simulink model "KF_Model_Div_Fixed"  (R2024b)
settings: Solver=FixedStepAuto  StartTime=0.0  StopTime=0.0025  FixedStep=5e-6  RelTol=1e-3
libraries: dspsrcs4 x3
settings Model: Creator=bzwan  LastModifiedBy=bzwan
settings OptimizationCC: UseDivisionForNetSlopeComputation=on
settings DebuggingCC: SignalRangeChecking=warning
settings HardwareCC: ProdBitPerPointer=32  ProdBitPerSizeT=32  ProdBitPerPtrDiffT=32  ProdLargestAtomicFloat=None  ProdIntDivRoundTo=Undefined  ProdEndianess=Unspecified  ProdWordSize=32  ProdHWDeviceType=ASIC/FPGA->ASIC/FPGA  TargetBitPerPointer=64  TargetBitPerSizeT=64  TargetBitPerPtrDiffT=64  TargetLongLongMode=on  TargetIntDivRoundTo=Zero  TargetEndianess=LittleEndian  TargetWordSize=64  TargetHWDeviceType=Custom Processor->MATLAB Host Computer  ProdEqTarget=off

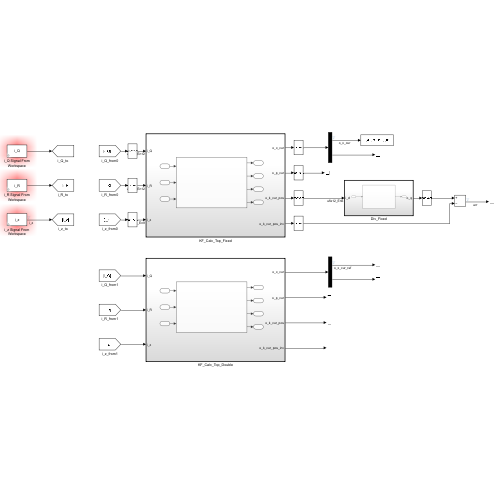
[thumbnail: Simulink's stored preview of the top-level diagram]
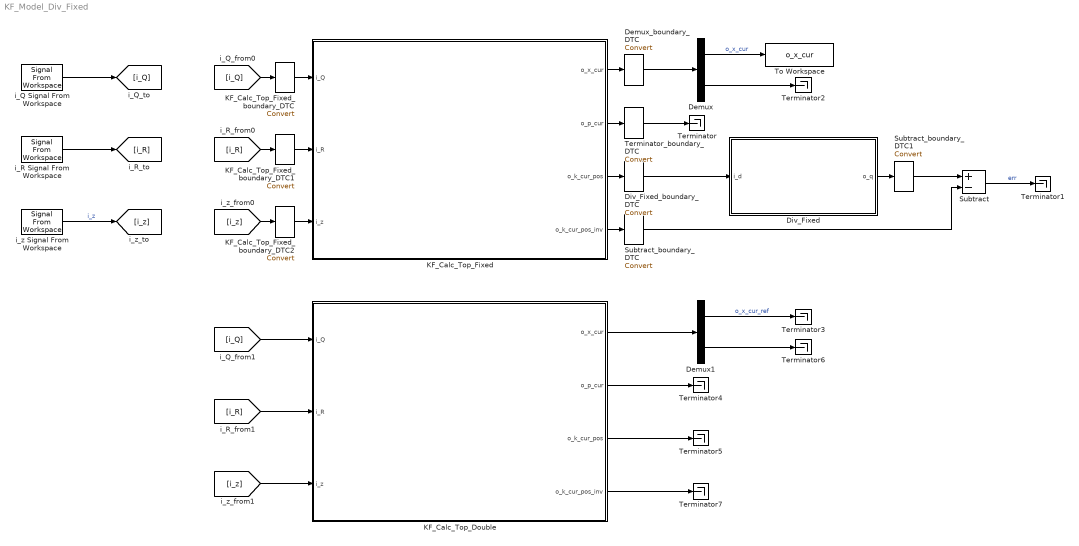
== system KF_Model_Div_Fixed ==
  Demux : Demux  Outputs=2
  Demux1 : Demux  Outputs=2
  Demux_boundary_DTC : DataTypeConversion
  Div_Fixed : Subsystem  TreatAsAtomicUnit=on  SystemSampleTime=1/10000
  Div_Fixed_boundary_DTC : DataTypeConversion
  KF_Calc_Top_Double : Subsystem  TreatAsAtomicUnit=on  SystemSampleTime=1/10000
  KF_Calc_Top_Fixed : Subsystem  TreatAsAtomicUnit=on  SystemSampleTime=1/10000
  KF_Calc_Top_Fixed_boundary_DTC : DataTypeConversion
  KF_Calc_Top_Fixed_boundary_DTC1 : DataTypeConversion
  KF_Calc_Top_Fixed_boundary_DTC2 : DataTypeConversion
  Subtract : Sum  Inputs=+-
  Subtract_boundary_DTC : DataTypeConversion
  Subtract_boundary_DTC1 : DataTypeConversion
  Terminator{,1..7} (8 alike) : Terminator
  Terminator_boundary_DTC : DataTypeConversion
  To Workspace : ToWorkspace  VariableName=o_x_cur  SaveFormat=Structure  SampleTime=-1
  i_Q Signal From Workspace : dspsrcs4/Signal From Workspace  X=i_Q  Ts=1/10000  nsamps=1  OutputAfterFinalValue=Cyclic repetition  ignoreOrWarnInputAndFrameLengths=off  OutputFrames=off
  i_R Signal From Workspace : dspsrcs4/Signal From Workspace  X=i_R  Ts=1/10000  nsamps=1  OutputAfterFinalValue=Cyclic repetition  ignoreOrWarnInputAndFrameLengths=off  OutputFrames=off
  i_z Signal From Workspace : dspsrcs4/Signal From Workspace  X=i_z  Ts=1/10000  nsamps=1  OutputAfterFinalValue=Cyclic repetition  ignoreOrWarnInputAndFrameLengths=off  OutputFrames=off
  wires:
  KF_Calc_Top_Double/1(o_x_cur) -> Demux1/1
  KF_Calc_Top_Double/2(o_p_cur) -> Terminator4/1
  KF_Calc_Top_Double/3(o_k_cur_pos) -> Terminator5/1
  i_Q Signal From Workspace/1 -> [i_Q]
  i_R Signal From Workspace/1 -> [i_R]
  i_z Signal From Workspace/1 -> [i_z]  "i_z"
  [i_z] -> KF_Calc_Top_Double/3(i_z)
  [i_R] -> KF_Calc_Top_Double/2(i_R)
  [i_Q] -> KF_Calc_Top_Double/1(i_Q)
  Demux/1 -> To Workspace/1  "o_x_cur"
  Demux/2 -> Terminator2/1
  Demux1/1 -> Terminator3/1  "o_x_cur_ref"
  Demux1/2 -> Terminator6/1
  Subtract/1 -> Terminator1/1  "err"
  KF_Calc_Top_Double/4(o_k_cur_pos_inv) -> Terminator7/1
  [i_Q] -> KF_Calc_Top_Fixed_boundary_DTC/1
  KF_Calc_Top_Fixed_boundary_DTC/1 -> KF_Calc_Top_Fixed/1(i_Q)
  [i_R] -> KF_Calc_Top_Fixed_boundary_DTC1/1
  KF_Calc_Top_Fixed_boundary_DTC1/1 -> KF_Calc_Top_Fixed/2(i_R)
  [i_z] -> KF_Calc_Top_Fixed_boundary_DTC2/1
  KF_Calc_Top_Fixed_boundary_DTC2/1 -> KF_Calc_Top_Fixed/3(i_z)
  KF_Calc_Top_Fixed/1(o_x_cur) -> Demux_boundary_DTC/1
  Demux_boundary_DTC/1 -> Demux/1
  KF_Calc_Top_Fixed/2(o_p_cur) -> Terminator_boundary_DTC/1
  Terminator_boundary_DTC/1 -> Terminator/1
  KF_Calc_Top_Fixed/3(o_k_cur_pos) -> Div_Fixed_boundary_DTC/1
  Div_Fixed_boundary_DTC/1 -> Div_Fixed/1(i_d)
  KF_Calc_Top_Fixed/4(o_k_cur_pos_inv) -> Subtract_boundary_DTC/1
  Subtract_boundary_DTC/1 -> Subtract/2
  Div_Fixed/1(o_q) -> Subtract_boundary_DTC1/1
  Subtract_boundary_DTC1/1 -> Subtract/1

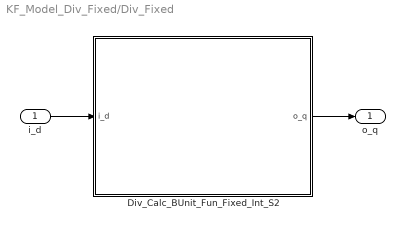
== system KF_Model_Div_Fixed/Div_Fixed ==
  i_d : Inport  OutDataTypeStr=fixdt(0,12,6)
  Div_Calc_BUnit_Fun_Fixed_Int_S2 : Subsystem  TreatAsAtomicUnit=on  Variant=on  VariantControlMode=label  VariantControl=Div_Calc_BUnit_Fun_Fixed_Int_S2  LabelModeActiveChoice=(default)
  o_q : Outport
  wires:
  i_d/1 -> Div_Calc_BUnit_Fun_Fixed_Int_S2/1(i_d)
  Div_Calc_BUnit_Fun_Fixed_Int_S2/1(o_q) -> o_q/1

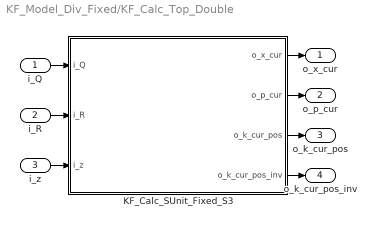
== system KF_Model_Div_Fixed/KF_Calc_Top_Double ==
  i_Q : Inport
  i_R : Inport  Port=2
  i_z : Inport  Port=3
  KF_Calc_SUnit_Fixed_S3 : MATLAB Function  TreatAsAtomicUnit=on
  o_x_cur : Outport
  o_p_cur : Outport  Port=2
  o_k_cur_pos : Outport  Port=3
  o_k_cur_pos_inv : Outport  Port=4
  wires:
  KF_Calc_SUnit_Fixed_S3/4(o_k_cur_pos_inv) -> o_k_cur_pos_inv/1
  KF_Calc_SUnit_Fixed_S3/2(o_p_cur) -> o_p_cur/1
  i_z/1 -> KF_Calc_SUnit_Fixed_S3/3(i_z)
  KF_Calc_SUnit_Fixed_S3/1(o_x_cur) -> o_x_cur/1
  i_Q/1 -> KF_Calc_SUnit_Fixed_S3/1(i_Q)
  i_R/1 -> KF_Calc_SUnit_Fixed_S3/2(i_R)
  KF_Calc_SUnit_Fixed_S3/3(o_k_cur_pos) -> o_k_cur_pos/1

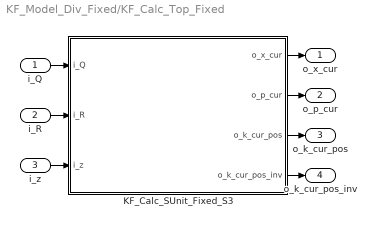
== system KF_Model_Div_Fixed/KF_Calc_Top_Fixed ==
  i_Q : Inport  OutDataTypeStr=fixdt(0,16,12)
  i_R : Inport  Port=2  OutDataTypeStr=fixdt(0,16,12)
  i_z : Inport  Port=3  OutDataTypeStr=fixdt(1,16,9)
  KF_Calc_SUnit_Fixed_S3 : Subsystem  TreatAsAtomicUnit=on  Variant=on  VariantControlMode=label  VariantControl=KF_Calc_SUnit_Fixed_S3  LabelModeActiveChoice=(default)
  o_x_cur : Outport
  o_p_cur : Outport  Port=2
  o_k_cur_pos : Outport  Port=3
  o_k_cur_pos_inv : Outport  Port=4
  wires:
  i_Q/1 -> KF_Calc_SUnit_Fixed_S3/1(i_Q)
  i_R/1 -> KF_Calc_SUnit_Fixed_S3/2(i_R)
  i_z/1 -> KF_Calc_SUnit_Fixed_S3/3(i_z)
  KF_Calc_SUnit_Fixed_S3/1(o_x_cur) -> o_x_cur/1
  KF_Calc_SUnit_Fixed_S3/2(o_p_cur) -> o_p_cur/1
  KF_Calc_SUnit_Fixed_S3/3(o_k_cur_pos) -> o_k_cur_pos/1
  KF_Calc_SUnit_Fixed_S3/4(o_k_cur_pos_inv) -> o_k_cur_pos_inv/1

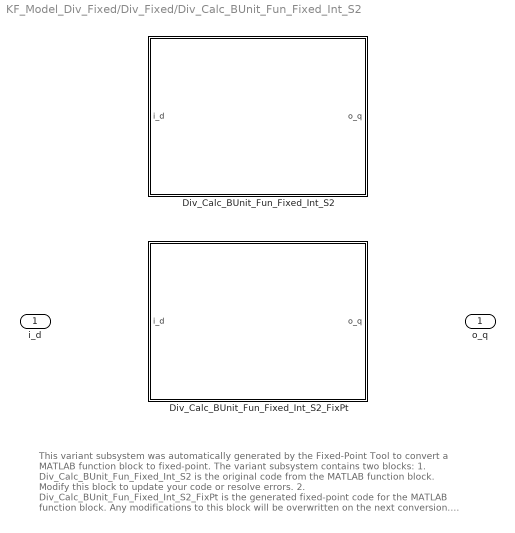
== system KF_Model_Div_Fixed/Div_Fixed/Div_Calc_BUnit_Fun_Fixed_Int_S2 ==
  note: This variant subsystem was automatically generated by the Fixed-Point Tool to convert a MATLAB function block to fixed-point.
      |
      | The variant subsystem contains two blocks:
      | 1. Div_Calc_BUnit_Fun_Fixed_Int_S2 is the original code from the MATLAB function block. Modify this block to update your code or resolve errors.
      |
      | 2. Div_Calc_BUnit_Fun_Fixed_Int_S2_FixPt is the generated fixed-point code for the MATLAB function block. Any modifications to this block will be overwritten on the next conversion.
      |
      | The Fixed-Point Tool will select an appropriate variant based on the Model Settings. Learn more.
  i_d : Inport
  Div_Calc_BUnit_Fun_Fixed_Int_S2 : MATLAB Function  TreatAsAtomicUnit=on  VariantControl=false()
  Div_Calc_BUnit_Fun_Fixed_Int_S2_FixPt : MATLAB Function  TreatAsAtomicUnit=on  VariantControl=(default)
  o_q : Outport

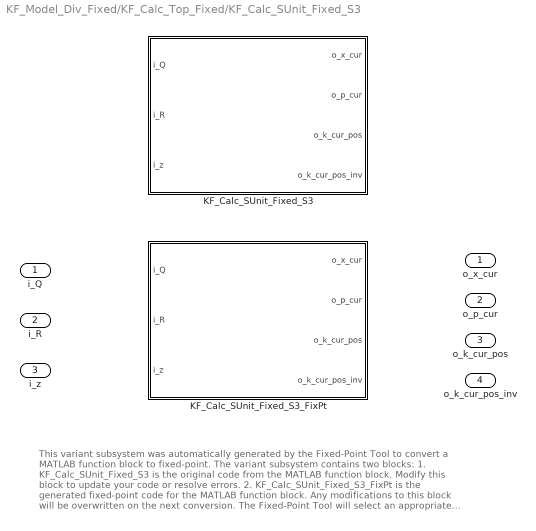
== system KF_Model_Div_Fixed/KF_Calc_Top_Fixed/KF_Calc_SUnit_Fixed_S3 ==
  note: This variant subsystem was automatically generated by the Fixed-Point Tool to convert a MATLAB function block to fixed-point.
      |
      | The variant subsystem contains two blocks:
      | 1. KF_Calc_SUnit_Fixed_S3 is the original code from the MATLAB function block. Modify this block to update your code or resolve errors.
      |
      | 2. KF_Calc_SUnit_Fixed_S3_FixPt is the generated fixed-point code for the MATLAB function block. Any modifications to this block will be overwritten on the next conversion.
      |
      | The Fixed-Point Tool will select an appropriate variant based on the Model Settings. Learn more.
  i_Q : Inport
  i_R : Inport  Port=2
  i_z : Inport  Port=3
  KF_Calc_SUnit_Fixed_S3 : MATLAB Function  TreatAsAtomicUnit=on  VariantControl=false()
  KF_Calc_SUnit_Fixed_S3_FixPt : MATLAB Function  TreatAsAtomicUnit=on  VariantControl=(default)
  o_x_cur : Outport
  o_p_cur : Outport  Port=2
  o_k_cur_pos : Outport  Port=3
  o_k_cur_pos_inv : Outport  Port=4

== matlab function KF_Model_Div_Fixed/KF_Calc_Top_Double/KF_Calc_SUnit_Fixed_S3 ==
  data: i_Q input; o_x_cur output; i_R input; i_z input; o_p_cur output; o_k_cur_pos output; o_k_cur_pos_inv output
function [o_x_cur, o_p_cur, o_k_cur_pos, o_k_cur_pos_inv]= KF_Calc_SUnit_Fixed_S3(i_Q, i_R, i_z) %#codegen
    
    % input is wire but hold as reg
    z = i_z;
    Q = i_Q;
    R = i_R;

    % reg define start
    persistent x_cur p_cur
    % reg define end
    
    if isempty(x_cur)
        x_cur = [0; 1];
    end

    if isempty(p_cur)
        p_cur = eye(2).*10;
    end

    % wire define start
    x_nxt_pre = zeros(2,1);
    x_nxt = zeros(2,1);
    p_nxt = zeros(2,2);
    k_cur_pre = zeros(2,1);
    k_cur_pos = zeros(1,1);
    k_cur_pos_inv = zeros(1,1);
    k_cur = zeros(2,1);
    x_cur_pos = zeros(1,1);
    p_cur_pre = zeros(2,2);
    % wire define end
    
    % predict
    x_nxt_pre(1,1) = (x_cur(1,1) + x_cur(2,1));
    x_nxt_pre(2,1) = x_cur(2,1);

    x_nxt(1,1) = x_nxt_pre(1,1);
    x_nxt(2,1) = x_nxt_pre(2,1);

    p_nxt(1,1) = (p_cur(1,1) + p_cur(2,1)) + ...
                 (p_cur(1,2) + p_cur(2,2)) + Q;
    p_nxt(1,2) = (p_cur(1,2) + p_cur(2,2));
    p_nxt(2,1) = (p_cur(2,1) + p_cur(2,2));
    p_nxt(2,2) = (p_cur(2,2) + Q);

    % update
    k_cur_pre(1,1) = p_nxt(1,1);
    k_cur_pre(2,1) = p_nxt(2,1);

    k_cur_pos(1,1) = (p_nxt(1,1) + R);

    if k_cur_pos(1,1) < .2e-1
        k_cur_pos(1,1) = .2e-1;
    end

    %%%%%%%%%%%%%%%%%%%%%%%%%%%%%%%%%%%%%%%%%%%%%%%%%%%%%%%
    o_k_cur_pos = k_cur_pos(1,1); % for fixed divider
    k_cur_pos_inv(1,1) = 1/k_cur_pos(1,1);
    o_k_cur_pos_inv = k_cur_pos_inv(1,1);
    %%%%%%%%%%%%%%%%%%%%%%%%%%%%%%%%%%%%%%%%%%%%%%%%%%%%%%%

    k_cur(1,1) = (k_cur_pre(1,1)*k_cur_pos_inv(1,1));
    k_cur(2,1) = (k_cur_pre(2,1)*k_cur_pos_inv(1,1));

    x_cur_pos(1,1) = (z(1,1) - x_nxt(1,1));

    x_cur(1,1) = (x_nxt(1,1) + (k_cur(1,1)*x_cur_pos(1,1)));
    x_cur(2,1) = (x_nxt(2,1) + (k_cur(2,1)*x_cur_pos(1,1)));

    p_cur_pre(1,1) = (1 - k_cur(1,1));
    p_cur_pre(1,2) = 0;
    p_cur_pre(2,1) = (0 - k_cur(2,1));
    p_cur_pre(2,2) = 1;

    p_cur(1,1) = (p_cur_pre(1,1)*p_nxt(1,1) + p_cur_pre(1,2)*p_nxt(2,1));
    p_cur(1,2) = (p_cur_pre(1,1)*p_nxt(1,2) + p_cur_pre(1,2)*p_nxt(2,2));
    p_cur(2,1) = (p_cur_pre(2,1)*p_nxt(1,1) + p_cur_pre(2,2)*p_nxt(2,1));
    p_cur(2,2) = (p_cur_pre(2,1)*p_nxt(1,2) + p_cur_pre(2,2)*p_nxt(2,2));

    o_x_cur = x_cur;
    o_p_cur = p_cur;
end

== matlab function KF_Model_Div_Fixed/KF_Calc_Top_Fixed/KF_Calc_SUnit_Fixed_S3/KF_Calc_SUnit_Fixed_S3 ==
  data: i_Q input; o_x_cur output; i_R input; i_z input; o_p_cur output; o_k_cur_pos output; o_k_cur_pos_inv output
function [o_x_cur, o_p_cur, o_k_cur_pos, o_k_cur_pos_inv]= KF_Calc_SUnit_Fixed_S3(i_Q, i_R, i_z) %#codegen
    
    % input is wire but hold as reg
    z = i_z;
    Q = i_Q;
    R = i_R;

    % reg define start
    persistent x_cur p_cur
    % reg define end
    
    if isempty(x_cur)
        x_cur = [0; 1];
    end

    if isempty(p_cur)
        p_cur = eye(2).*10;
    end

    % wire define start
    x_nxt_pre = zeros(2,1);
    x_nxt = zeros(2,1);
    p_nxt = zeros(2,2);
    k_cur_pre = zeros(2,1);
    k_cur_pos = zeros(1,1);
    k_cur_pos_inv = zeros(1,1);
    k_cur = zeros(2,1);
    x_cur_pos = zeros(1,1);
    p_cur_pre = zeros(2,2);
    % wire define end
    
    % predict
    x_nxt_pre(1,1) = (x_cur(1,1) + x_cur(2,1));
    x_nxt_pre(2,1) = x_cur(2,1);

    x_nxt(1,1) = x_nxt_pre(1,1);
    x_nxt(2,1) = x_nxt_pre(2,1);

    p_nxt(1,1) = (p_cur(1,1) + p_cur(2,1)) + ...
                 (p_cur(1,2) + p_cur(2,2)) + Q;
    p_nxt(1,2) = (p_cur(1,2) + p_cur(2,2));
    p_nxt(2,1) = (p_cur(2,1) + p_cur(2,2));
    p_nxt(2,2) = (p_cur(2,2) + Q);

    % update
    k_cur_pre(1,1) = p_nxt(1,1);
    k_cur_pre(2,1) = p_nxt(2,1);

    k_cur_pos(1,1) = (p_nxt(1,1) + R);

    if k_cur_pos(1,1) < .2e-1
        k_cur_pos(1,1) = .2e-1;
    end

    %%%%%%%%%%%%%%%%%%%%%%%%%%%%%%%%%%%%%%%%%%%%%%%%%%%%%%%
    o_k_cur_pos = k_cur_pos(1,1); % for fixed divider
    k_cur_pos_inv(1,1) = 1/k_cur_pos(1,1);
    o_k_cur_pos_inv = k_cur_pos_inv(1,1);
    %%%%%%%%%%%%%%%%%%%%%%%%%%%%%%%%%%%%%%%%%%%%%%%%%%%%%%%

    k_cur(1,1) = (k_cur_pre(1,1)*k_cur_pos_inv(1,1));
    k_cur(2,1) = (k_cur_pre(2,1)*k_cur_pos_inv(1,1));

    x_cur_pos(1,1) = (z(1,1) - x_nxt(1,1));

    x_cur(1,1) = (x_nxt(1,1) + (k_cur(1,1)*x_cur_pos(1,1)));
    x_cur(2,1) = (x_nxt(2,1) + (k_cur(2,1)*x_cur_pos(1,1)));

    p_cur_pre(1,1) = (1 - k_cur(1,1));
    p_cur_pre(1,2) = 0;
    p_cur_pre(2,1) = (0 - k_cur(2,1));
    p_cur_pre(2,2) = 1;

    p_cur(1,1) = (p_cur_pre(1,1)*p_nxt(1,1) + p_cur_pre(1,2)*p_nxt(2,1));
    p_cur(1,2) = (p_cur_pre(1,1)*p_nxt(1,2) + p_cur_pre(1,2)*p_nxt(2,2));
    p_cur(2,1) = (p_cur_pre(2,1)*p_nxt(1,1) + p_cur_pre(2,2)*p_nxt(2,1));
    p_cur(2,2) = (p_cur_pre(2,1)*p_nxt(1,2) + p_cur_pre(2,2)*p_nxt(2,2));

    o_x_cur = x_cur;
    o_p_cur = p_cur;
end

== matlab function KF_Model_Div_Fixed/KF_Calc_Top_Fixed/KF_Calc_SUnit_Fixed_S3/KF_Calc_SUnit_Fixed_S3_FixPt ==
  settings: fimath=|
      | fimath('RoundingMethod', 'Nearest',...
      | 'OverflowAction', 'Saturate',...
      | 'ProductMode','FullPrecision',...
      | 'SumMode','FullPrecision')
  data: i_Q input; o_x_cur output; i_R input; i_z input; o_p_cur output; o_k_cur_pos output; o_k_cur_pos_inv output
%auto-generated
function [o_x_cur, o_p_cur, o_k_cur_pos, o_k_cur_pos_inv]= KF_Calc_SUnit_Fixed_S3_fixpt(i_Q, i_R, i_z) %#codegen
    
    % input is wire but hold as reg
    fm = get_fimath();
    i_Q = fi(i_Q, 0, 16, 12, fm);
    i_R = fi(i_R, 0, 16, 12, fm);
    i_z = fi(i_z, 1, 16, 9, fm);

    z = fi(i_z, 1, 16, 9, fm);
    Q = fi(i_Q, 0, 16, 12, fm);
    R = fi(i_R, 0, 16, 12, fm);

    % reg define start
    persistent x_cur p_cur
    % reg define end
    
    if isempty(x_cur)
        x_cur = fi([0; 1], 1, 18, 10, fm);
    end

    if isempty(p_cur)
        p_cur = fi(eye(2).*10, 0, 16, 11, fm);
    end

    % wire define start
    x_nxt_pre = fi(zeros(2,1), 1, 18, 10, fm);
    x_nxt = fi(zeros(2,1), 1, 18, 10, fm);
    p_nxt = fi(zeros(2,2), 0, 10, 4, fm);
    k_cur_pre = fi(zeros(2,1), 0, 12, 6, fm);
    k_cur_pos = fi(zeros(1,1), 0, 12, 6, fm);
    k_cur_pos_inv = fi(zeros(1,1), 0, 12, 14, fm);
    k_cur = fi(zeros(2,1), 0, 12, 12, fm);
    x_cur_pos = fi(zeros(1,1), 1, 16, 8, fm);
    p_cur_pre = fi(zeros(2,2), 1, 15, 13, fm);
    % wire define end
    
    % predict
    x_nxt_pre(1,1) = (x_cur(1,1) + x_cur(2,1));
    x_nxt_pre(2,1) = x_cur(2,1);

    x_nxt(1,1) = x_nxt_pre(1,1);
    x_nxt(2,1) = x_nxt_pre(2,1);

    p_nxt(1,1) = removefimath((p_cur(1,1) + p_cur(2,1)) + ...
                 (p_cur(1,2) + p_cur(2,2))) + Q;
    p_nxt(1,2) = (p_cur(1,2) + p_cur(2,2));
    p_nxt(2,1) = (p_cur(2,1) + p_cur(2,2));
    p_nxt(2,2) = (fi(removefimath(p_cur(2,2)) + Q, fm));

    % update
    k_cur_pre(1,1) = p_nxt(1,1);
    k_cur_pre(2,1) = p_nxt(2,1);

    k_cur_pos(1,1) = (fi(removefimath(p_nxt(1,1)) + R, fm));

    if k_cur_pos(1,1) < fi(.2e-1, 0, 16, 21, fm)
        k_cur_pos(1,1) = .2e-1;
    end

    %%%%%%%%%%%%%%%%%%%%%%%%%%%%%%%%%%%%%%%%%%%%%%%%%%%%%%%
    o_k_cur_pos = fi(k_cur_pos(1,1), 0, 12, 6, fm); % for fixed divider
    k_cur_pos_inv(1,1) = fi_div(fi(1, 0, 1, 0, fm), k_cur_pos(1,1));
    o_k_cur_pos_inv = fi(k_cur_pos_inv(1,1), 0, 12, 14, fm);
    %%%%%%%%%%%%%%%%%%%%%%%%%%%%%%%%%%%%%%%%%%%%%%%%%%%%%%%

    k_cur(1,1) = (k_cur_pre(1,1)*k_cur_pos_inv(1,1));
    k_cur(2,1) = (k_cur_pre(2,1)*k_cur_pos_inv(1,1));

    x_cur_pos(1,1) = (fi_signed(z(1,1)) - x_nxt(1,1));

    x_cur(1,1) = (x_nxt(1,1) + (k_cur(1,1)*x_cur_pos(1,1)));
    x_cur(2,1) = (x_nxt(2,1) + (k_cur(2,1)*x_cur_pos(1,1)));

    p_cur_pre(1,1) = (fi_signed(fi(1, 0, 1, 0, fm)) - k_cur(1,1));
    p_cur_pre(1,2) = 0;
    p_cur_pre(2,1) = (fi_signed(fi(0, 0, 1, 0, fm)) - k_cur(2,1));
    p_cur_pre(2,2) = 1;

    p_cur(1,1) = (p_cur_pre(1,1)*p_nxt(1,1) + p_cur_pre(1,2)*p_nxt(2,1));
    p_cur(1,2) = (p_cur_pre(1,1)*p_nxt(1,2) + p_cur_pre(1,2)*p_nxt(2,2));
    p_cur(2,1) = (p_cur_pre(2,1)*p_nxt(1,1) + p_cur_pre(2,2)*p_nxt(2,1));
    p_cur(2,2) = (p_cur_pre(2,1)*p_nxt(1,2) + p_cur_pre(2,2)*p_nxt(2,2));

    o_x_cur = fi(x_cur, 1, 18, 10, fm);
    o_p_cur = fi(p_cur, 0, 16, 11, fm);
end



function ntype = divideType(a,b)
    coder.inline( 'always' );
    nt1 = numerictype( a );
    nt2 = numerictype( b );
    maxFL = max( [ min( nt1.WordLength, nt1.FractionLength ), min( nt2.WordLength, nt2.FractionLength ) ] );
    FL = max( maxFL, 24 );
    extraBits = (FL - maxFL);
    WL = nt1.WordLength + nt2.WordLength;
    WL = min( WL, 124 );
    if (WL + extraBits)<64
        ntype = numerictype( nt1.Signed || nt2.Signed, WL + extraBits, FL );
    else
        ntype = numerictype( nt1.Signed || nt2.Signed, WL, FL );
    end
end


function c = fi_div(a,b)
    coder.inline( 'always' );
    a1 = fi( a, 'RoundMode', 'fix' );
    b1 = fi( b, 'RoundMode', 'fix' );
    nType = divideType( a1, b1 );
    if isfi( a ) && isfi( b ) && isscalar( b )
        c1 = divide( nType, a1, b1 );
        c = fi( c1, numerictype( c1 ), fimath( a ) );
    else
        c = fi( a / b, nType );
    end
end


function y = fi_signed(a)
    coder.inline( 'always' );
    if isfi( a ) && ~(issigned( a ))
        nt = numerictype( a );
        new_nt = numerictype( 1, nt.WordLength + 1, nt.FractionLength );
        y = fi( a, new_nt, fimath( a ) );
    else
        y = a;
    end
end

function fm = get_fimath()
	fm = fimath('RoundingMethod', 'Nearest',...
	     'OverflowAction', 'Saturate',...
	     'ProductMode','FullPrecision',...
	     'SumMode','FullPrecision');
end

== matlab function KF_Model_Div_Fixed/Div_Fixed/Div_Calc_BUnit_Fun_Fixed_Int_S2/Div_Calc_BUnit_Fun_Fixed_Int_S2 ==
  data: i_d input; o_q output
function o_q = Div_Calc_BUnit_Fun_Fixed_Int_S2(i_d) %#codegen

    % input is wire
    abs_z = 1;
    abs_d = i_d;

    % reg define start
    loop_cnt = 0;
    iter_cnt = 8;
    z = zeros(1,iter_cnt);
    d = zeros(1,iter_cnt);
    % reg define end

    % step 1: normal ensure d less than 2^-1
    loop_abs = abs_d*64; % 12,6
    bit_sel = bitget(double(loop_abs), 1:16, 'uint16');
    if bit_sel(12) == 1
        loop_cnt = 6;
    elseif bit_sel(11) == 1
        loop_cnt = 5;
    elseif bit_sel(10) == 1
        loop_cnt = 4;
    elseif bit_sel(9) == 1
        loop_cnt = 3;
    elseif bit_sel(8) == 1
        loop_cnt = 2;
    elseif bit_sel(7) == 1
        loop_cnt = 1;
    elseif bit_sel(6) == 1
        loop_cnt = 0;
    elseif bit_sel(5) == 1
        loop_cnt = -1;
    elseif bit_sel(4) == 1
        loop_cnt = -2;
    elseif bit_sel(3) == 1
        loop_cnt = -3;
    elseif bit_sel(2) == 1
        loop_cnt = -4;
    elseif bit_sel(1) == 1
        loop_cnt = -5;
    else
        loop_cnt = 0;
    end
    
    % step 2: init
    z(1,1) = abs_z;
    
    tmp_d = abs_d;
    if loop_cnt >= 0
        tmp_d = bitsra(tmp_d, abs(loop_cnt));
    else
        tmp_d = bitsll(tmp_d, abs(loop_cnt));
    end

    d(1,1) = tmp_d;
    
    % step 3: iter
    mul_factor = (2 - d(1,1));
    for idx_i = 2:iter_cnt
        z(1,idx_i) = z(1,idx_i-1) * mul_factor;
        d(1,idx_i) = d(1,idx_i-1) * mul_factor;
        mul_factor = (2 - d(1,idx_i));
    end
    
    % step 4: recover
    tmp_z = z(1,iter_cnt);
    if loop_cnt >= 0
        tmp_z = bitsra(tmp_z, abs(loop_cnt));
    else
        tmp_z = bitsll(tmp_z, abs(loop_cnt));
    end
    
    q = tmp_z;

    o_q = q;
end

== matlab function KF_Model_Div_Fixed/Div_Fixed/Div_Calc_BUnit_Fun_Fixed_Int_S2/Div_Calc_BUnit_Fun_Fixed_Int_S2_FixPt ==
  settings: fimath=|
      | fimath('RoundingMethod', 'Nearest',...
      | 'OverflowAction', 'Saturate',...
      | 'ProductMode','FullPrecision',...
      | 'SumMode','FullPrecision')
  data: i_d input; o_q output
%auto-generated
function o_q = Div_Calc_BUnit_Fun_Fixed_Int_S2_fixpt(i_d) %#codegen

    % input is wire
    fm = get_fimath();
    i_d = fi(i_d, 0, 12, 6, fm);

    abs_z = fi(1, 0, 12, 11, fm);
    abs_d = fi(i_d, 0, 12, 6, fm);

    % reg define start
    loop_cnt = fi(0, 0, 12, 9, fm);
    iter_cnt = fi(8, 0, 12, 8, fm);
    z = fi(zeros(1,fi_toint(iter_cnt)), 0, 12, 10, fm);
    d = fi(zeros(1,fi_toint(iter_cnt)), 0, 12, 11, fm);
    % reg define end

    % step 1: normal ensure d less than 2^-1
    loop_abs = fi(abs_d*removefimath(fi(64, 0, 7, 0, fm)), 0, 12, 0, fm); % 12,6
    bit_sel = fi(bitget(double(loop_abs), 1:16, 'uint16'), 0, 12, 11, fm);
    if bit_sel(12) == fi(1, 0, 1, 0, fm)
        loop_cnt(:) = 6;
    elseif bit_sel(11) == fi(1, 0, 1, 0, fm)
        loop_cnt(:) = 5;
    elseif bit_sel(10) == fi(1, 0, 1, 0, fm)
        loop_cnt(:) = 4;
    elseif bit_sel(9) == fi(1, 0, 1, 0, fm)
        loop_cnt(:) = 3;
    elseif bit_sel(8) == fi(1, 0, 1, 0, fm)
        loop_cnt(:) = 2;
    elseif bit_sel(7) == fi(1, 0, 1, 0, fm)
        loop_cnt(:) = 1;
    elseif bit_sel(6) == fi(1, 0, 1, 0, fm)
        loop_cnt(:) = 0;
    elseif bit_sel(5) == fi(1, 0, 1, 0, fm)
        loop_cnt(:) = -1;
    elseif bit_sel(4) == fi(1, 0, 1, 0, fm)
        loop_cnt(:) = -2;
    elseif bit_sel(3) == fi(1, 0, 1, 0, fm)
        loop_cnt(:) = -3;
    elseif bit_sel(2) == fi(1, 0, 1, 0, fm)
        loop_cnt(:) = -4;
    elseif bit_sel(1) == fi(1, 0, 1, 0, fm)
        loop_cnt(:) = -5;
    else
        loop_cnt(:) = 0;
    end
    
    % step 2: init
    z(1,1) = abs_z;
    
    tmp_d = fi(abs_d, 0, 12, 6, fm);
    if loop_cnt >= fi(0, 0, 1, 0, fm)
        tmp_d(:) = bitsra(tmp_d, fi_toint(abs(loop_cnt)));
    else
        tmp_d(:) = bitsll(tmp_d, fi_toint(abs(loop_cnt)));
    end

    d(1,1) = tmp_d;
    
    % step 3: iter
    mul_factor = fi((fi_signed(fi(2, 0, 2, 0, fm)) - d(1,1)), 0, 12, 11, fm);
    for idx_i = fi(2, 0, 2, 0, fm):iter_cnt
        z(1,idx_i) = removefimath(z(1,fi(idx_i-removefimath(fi(1, 0, 1, 0, fm)), fm))) * mul_factor;
        d(1,idx_i) = removefimath(d(1,fi(idx_i-removefimath(fi(1, 0, 1, 0, fm)), fm))) * mul_factor;
        mul_factor(:) = (fi_signed(fi(2, 0, 2, 0, fm)) - d(1,idx_i));
    end
    
    % step 4: recover
    tmp_z = fi(z(1,iter_cnt), 0, 12, 10, fm);
    if loop_cnt >= fi(0, 0, 1, 0, fm)
        tmp_z(:) = bitsra(tmp_z, fi_toint(abs(loop_cnt)));
    else
        tmp_z(:) = bitsll(tmp_z, fi_toint(abs(loop_cnt)));
    end
    
    q = fi(tmp_z, 0, 12, 14, fm);

    o_q = fi(q, 0, 12, 14, fm);
end



function y = fi_signed(a)
    coder.inline( 'always' );
    if isfi( a ) && ~(issigned( a ))
        nt = numerictype( a );
        new_nt = numerictype( 1, nt.WordLength + 1, nt.FractionLength );
        y = fi( a, new_nt, fimath( a ) );
    else
        y = a;
    end
end


function y = fi_toint(u)
    coder.inline( 'always' );
    if isfi( u )
        nt = numerictype( u );
        s = nt.SignednessBool;
        wl = nt.WordLength;
        y = int32( fi( u, s, wl, 0, hdlfimath ) );
    else
        y = int32( u );
    end
end

function fm = get_fimath()
	fm = fimath('RoundingMethod', 'Nearest',...
	     'OverflowAction', 'Saturate',...
	     'ProductMode','FullPrecision',...
	     'SumMode','FullPrecision');
end
